simulink model "aai"  (R2020a)
settings: Solver=FixedStepAuto  StartTime=0.0  StopTime=10.0  FixedStep=1e-3  RelTol=1e-3  EnableMultiTasking=on
undefined symbols (not defined in the file): D0, D10, D11, D12, D13, D2, D4, D5, D6, D7, D8, D9, PTA0, PTA2, PTB23, PTB9, PTC16, PTC2, PTC3, PTC4, PTD0, PTD1, PTD2, PTD3
libraries: frdmk64flib x12
settings Model: ExtModeTrigDuration=5  Creator=raymo  LastModifiedBy=raymo
settings OptimizationCC: EnhancedBackFolding=on  PassReuseOutputArgsAs=Individual arguments  ZeroExternalMemoryAtStartup=off  ZeroInternalMemoryAtStartup=off  MaxStackSize=64  OptimizeBlockOrder=speed  DifferentSizesBufferReuse=on  OptimizationCustomize=off  EfficientTunableParamExpr=on
settings DebuggingCC: ParameterTunabilityLossMsg=error
settings HardwareCC: ProdBitPerPointer=32  ProdBitPerSizeT=32  ProdBitPerPtrDiffT=32  ProdLargestAtomicInteger=Long  ProdLargestAtomicFloat=Double  ProdWordSize=32  ProdHWDeviceType=ARM Compatible->ARM Cortex
settings SFSimCC: MATLABDynamicMemAlloc=off
settings RTWCC: SystemTargetFile=ert.tlc  HardwareBoard=NXP FRDM-K64F  TemplateMakefile=ert_default_tmf  Toolchain=GNU Tools for ARM Embedded Processors
settings CodeAppCC: ForceParamTrailComments=on  IgnoreCustomStorageClasses=off  OperatorAnnotations=on  SimulinkDataObjDesc=on  SFDataObjDesc=on  InsertBlockDesc=on

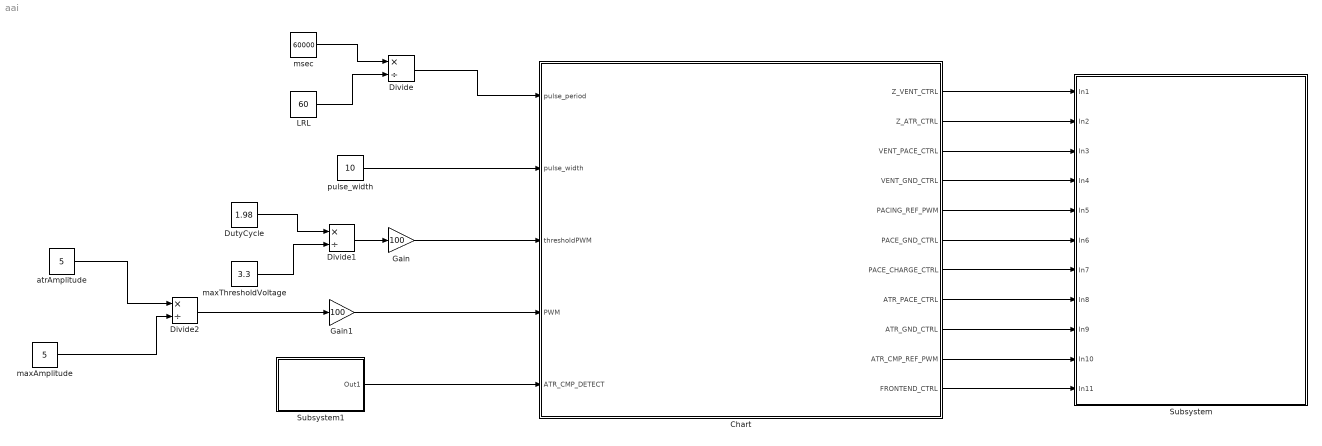
== system aai ==
  Chart : Stateflow chart  TreatAsAtomicUnit=on
  Divide : Product  Inputs=*/
  Divide1 : Product  Inputs=*/
  Divide2 : Product  Inputs=*/
  DutyCycle : Constant  Value=1.98
  Gain : Gain  Gain=100
  Gain1 : Gain  Gain=100
  LRL : Constant  Value=60
  Subsystem : Subsystem
  Subsystem1 : Subsystem
  atrAmplitude : Constant  Value=5
  maxAmplitude : Constant  Value=5
  maxThresholdVoltage : Constant  Value=3.3
  msec : Constant  Value=60000
  pulse_width : Constant  Value=10
  wires:
  Divide1/1 -> Gain/1
  pulse_width/1 -> Chart/2(pulse_width)
  Gain1/1 -> Chart/4(PWM)
  msec/1 -> Divide/1
  LRL/1 -> Divide/2
  Divide/1 -> Chart/1(pulse_period)
  Chart/1(Z_VENT_CTRL) -> Subsystem/1(In1)
  Chart/2(Z_ATR_CTRL) -> Subsystem/2(In2)
  Chart/3(VENT_PACE_CTRL) -> Subsystem/3(In3)
  Chart/4(VENT_GND_CTRL) -> Subsystem/4(In4)
  Chart/5(PACING_REF_PWM) -> Subsystem/5(In5)
  Chart/6(PACE_GND_CTRL) -> Subsystem/6(In6)
  Chart/7(PACE_CHARGE_CTRL) -> Subsystem/7(In7)
  Chart/8(ATR_PACE_CTRL) -> Subsystem/8(In8)
  Chart/9(ATR_GND_CTRL) -> Subsystem/9(In9)
  Chart/10(ATR_CMP_REF_PWM) -> Subsystem/10(In10)
  Chart/11(FRONTEND_CTRL) -> Subsystem/11(In11)
  DutyCycle/1 -> Divide1/1
  maxThresholdVoltage/1 -> Divide1/2
  maxAmplitude/1 -> Divide2/2
  atrAmplitude/1 -> Divide2/1
  Gain/1 -> Chart/3(thresholdPWM)
  Divide2/1 -> Gain1/1
  Subsystem1/1(Out1) -> Chart/5(ATR_CMP_DETECT)

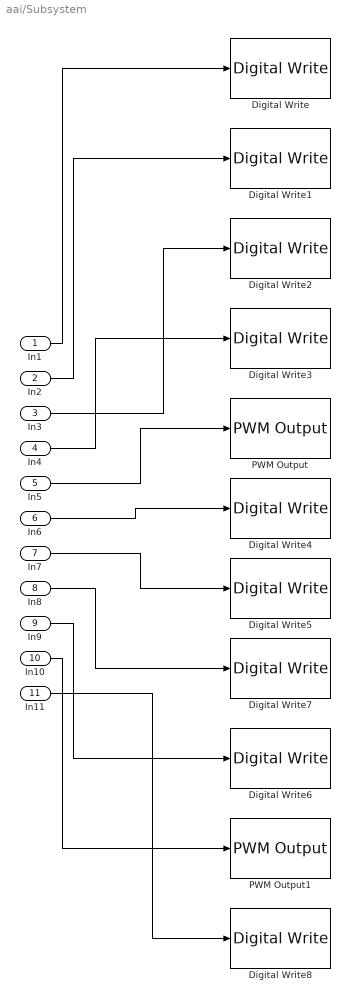
== system aai/Subsystem ==
  In1 : Inport
  In2 : Inport  Port=2
  In3 : Inport  Port=3
  In4 : Inport  Port=4
  In5 : Inport  Port=5
  In6 : Inport  Port=6
  In7 : Inport  Port=7
  In8 : Inport  Port=8
  In9 : Inport  Port=9
  In10 : Inport  Port=10
  In11 : Inport  Port=11
  Digital Write : frdmk64flib/Digital Write  Whichpin=PTC3 (D7)
  Digital Write1 : frdmk64flib/Digital Write  Whichpin=PTB23 (D4)
  Digital Write2 : frdmk64flib/Digital Write  Whichpin=PTC4 (D9)
  Digital Write3 : frdmk64flib/Digital Write  Whichpin=PTD3 (D12)
  Digital Write4 : frdmk64flib/Digital Write  Whichpin=PTD0 (D10)
  Digital Write5 : frdmk64flib/Digital Write  Whichpin=PTB9 (D2)
  Digital Write6 : frdmk64flib/Digital Write  Whichpin=PTD2 (D11)
  Digital Write7 : frdmk64flib/Digital Write  Whichpin=PTA0 (D8)
  Digital Write8 : frdmk64flib/Digital Write  Whichpin=PTD1 (D13)
  PWM Output : frdmk64flib/PWM Output  Whichpin=PTA2 (D5)  InitialFrequency=2000  InitialDutyCycle=50
  PWM Output1 : frdmk64flib/PWM Output  Whichpin=PTC2 (D6)  InitialFrequency=2000  InitialDutyCycle=50
  wires:
  In5/1 -> PWM Output/1
  In3/1 -> Digital Write2/1
  In1/1 -> Digital Write/1
  In4/1 -> Digital Write3/1
  In8/1 -> Digital Write7/1
  In9/1 -> Digital Write6/1
  In7/1 -> Digital Write5/1
  In2/1 -> Digital Write1/1
  In11/1 -> Digital Write8/1
  In10/1 -> PWM Output1/1
  In6/1 -> Digital Write4/1

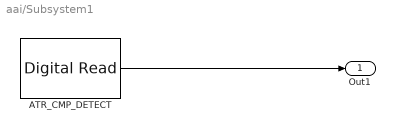
== system aai/Subsystem1 ==
  ATR_CMP_DETECT : frdmk64flib/Digital Read  Whichpin=PTC16 (D0)  SampleTime=-1
  Out1 : Outport
  wires:
  ATR_CMP_DETECT/1 -> Out1/1

== stateflow chart aai/Chart ==
  state Idle
    entry:
    %Set threshold
    ATR_CMP_REF_PWM = thresholdPWM;
    FRONTEND_CTRL = 1;
  state AVpacing
    entry:
    PACE_CHARGE_CTRL = 0;
    PACE_GND_CTRL = 1;
    ATR_PACE_CTRL = 1;
    ATR_GND_CTRL = 0;
    Z_ATR_CTRL = 0;
    Z_VENT_CTRL = 0;
    VENT_GND_CTRL = 0;
    VENT_PACE_CTRL = 0;
    PACING_REF_PWM = PWM;
  state ChargeDischarge
    entry:
    %C22
    ATR_PACE_CTRL = 0;
    VENT_PACE_CTRL = 0;
    PACING_REF_PWM = PWM;
    PACE_CHARGE_CTRL = 1;
    %C21
    PACE_GND_CTRL = 1;
    VENT_PACE_CTRL = 0;
    Z_ATR_CTRL = 0;
    Z_VENT_CTRL = 0;
    ATR_GND_CTRL = 1;
    VENT_GND_CTRL = 0;
  (default) -> Idle
  Idle -> ChargeDischarge
  ChargeDischarge -> ChargeDischarge [order 1] : after(pulse_width,msec)[ATR_CMP_DETECT == 1]
  ChargeDischarge -> AVpacing [order 2] : [after(pulse_period-pulse_width,msec)]
  AVpacing -> ChargeDischarge : [after(pulse_width, msec)]
  data: pulse_period input; pulse_width input; thresholdPWM input; PWM input; Z_VENT_CTRL output; Z_ATR_CTRL output; VENT_PACE_CTRL output; VENT_GND_CTRL output; PACING_REF_PWM output; PACE_GND_CTRL output; PACE_CHARGE_CTRL output; ATR_PACE_CTRL output; ATR_GND_CTRL output; ATR_CMP_REF_PWM output; ATR_CMP_DETECT input; FRONTEND_CTRL output
